simulink model "sgMdl_IO424_LVDTMeasurementTest"  (R2024b)
settings: Solver=FixedStepAuto  StartTime=0.0  StopTime=inf  RelTol=1e-3
model workspace (MAT data in the model file):
  La_ratio = 0.5
libraries: dspsrcs4 x3, speedgoatlib_IO424 x2, speedgoatlib_IO107 x1
Description:
  | IO424 - LVDT Measurement
settings Model: ModifiedByFormat=Speedgoat  SimulationMode=external  ExtModeEnableFloating=off  Creator=Speedgoat  LastModifiedBy=Speedgoat
settings SolverCC: ConcurrentTasks=on  PositivePriorityOrder=on
settings OptimizationCC: BlockReduction=off  OptimizeBlockIOStorage=off
settings DebuggingCC: TasksWithSamePriorityMsg=none
settings HardwareCC: ProdBitPerLong=64  ProdLongLongMode=on  ProdHWDeviceType=Intel->x86-64 (Linux 64)
settings RTWCC: Description=Speedgoat Real-Time Target Machine  SystemTargetFile=speedgoat.tlc  TemplateMakefile=slrealtime_default_tmf  Toolchain=Simulink Real-Time Toolchain  BuildConfiguration=Faster Runs  TargetLang=C++
settings SimulinkRealTimeTargetCC: SubcomponentCodeInterfacePackaging=Reusable function  InstructionSetFMA=off  LogToMDFFile=off  SLRTLogLevel=debug  SLRTFileLogMaxRuns=10
settings ConfigComp: CovBoundaryAbsTol=1.0e-5

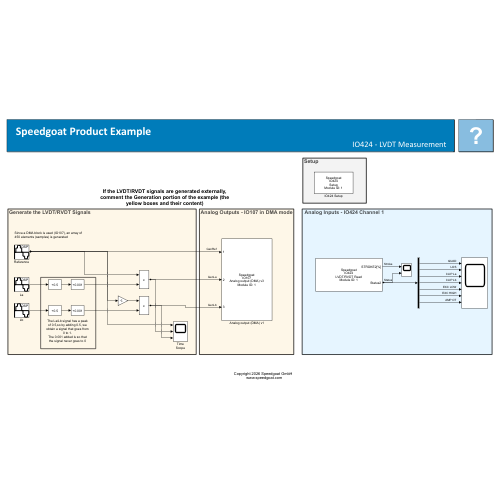
[thumbnail: Simulink's stored preview of the top-level diagram]
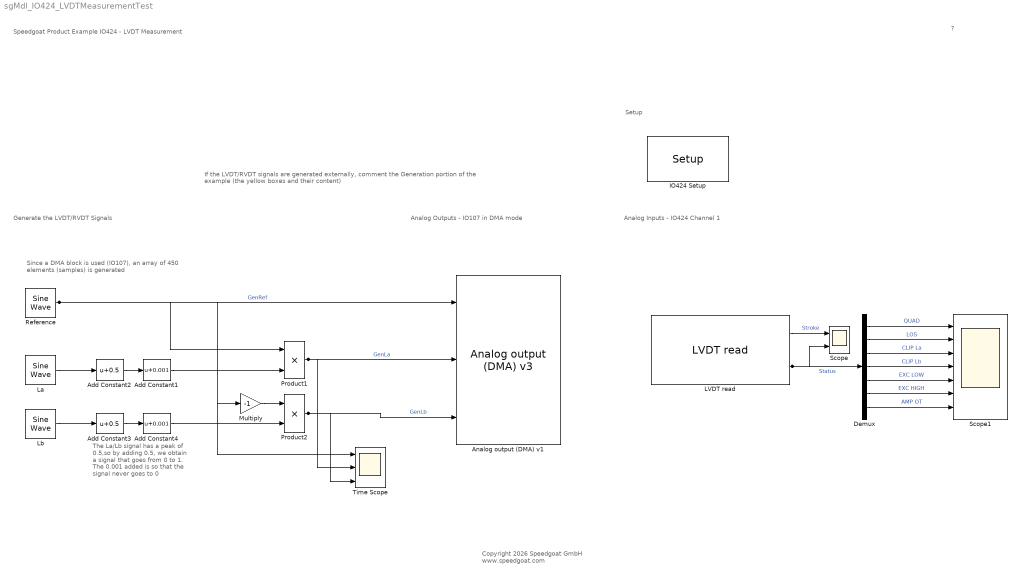
== system sgMdl_IO424_LVDTMeasurementTest ==
  note: The La/Lb signal has a peak
      | of 0.5,so by adding 0.5, we
      | obtain a signal that goes from
      | 0 to 1.
      | The 0.001 added is so that
      | the signal never goes to 0
  note: If the LVDT/RVDT signals are generated externally, comment the Generation portion of the example (the yellow boxes and their content)
  note: Analog Outputs - IO107 in DMA mode
  note: Analog Inputs - IO424 Channel 1
  note: Generate the LVDT/RVDT Signals
  note: Setup
  note: Since a DMA block is used (IO107), an array of
      | 450 elements (samples) is generated
  note: Speedgoat Product Example
      | IO424 - LVDT Measurement
  note: ?
  note: Copyright 2026 Speedgoat GmbH
      |  www.speedgoat.com
  Add Constant1 : Bias  Bias=0.001  SaturateOnIntegerOverflow=off
  Add Constant2 : Bias  Bias=0.5  SaturateOnIntegerOverflow=off
  Add Constant3 : Bias  Bias=0.5  SaturateOnIntegerOverflow=off
  Add Constant4 : Bias  Bias=0.001  SaturateOnIntegerOverflow=off
  Analog output (DMA) v1 : speedgoatlib_IO107/Analog output (DMA) v3  id=1  slot=-1  channel_str=[11 1 10]  range=+-10.0  parInit_str=[0]  parReset_str=[1]  autocal=on  gsense=off  clksrc=Internal  syncmode=Async (replay function)  extsync=LVDS  framesize_str=450  samplerate_str=450e3  sampletime_str=-1
      settings: SourceProductName=IO107
  Demux : Demux  Outputs=7
  IO424 Setup : speedgoatlib_IO424/Setup  parId=1  parModType=IO424-R (no Synchro)  parPciSlot=-1  parChConf1=LVDT/RVDT Ratiometric (6-wires)  parChConf2=Disabled  parChConf3=Disabled  parChConf4=Disabled  parPosRdcUnit=Radiants  parCombRdcCh12=on  parCombRdcCh34=on  parChRdcRange1=7.07 Vrms  parChRdcRange2=14.14 Vrms  parChRdcRange3=14.14 Vrms  parChRdcRange4=14.14 Vrms  parPosSynchroUnit=Radiants  parCombSynchroCh34=on  parChSynchroRange3=28 Vrms  parChSynchroRange4=28 Vrms  parCombLvdtCh12=on  parCombLvdtCh34=on  parLvdtRange1A=7.07 Vrms  parLvdtRange1B=7.07 Vrms  parLvdtRange2A=7.07 Vrms  parLvdtRange2B=14.14 Vrms  parLvdtRange3A=7.07 Vrms  parLvdtRange3B=7.07 Vrms  parLvdtRange4A=7.07 Vrms  parLvdtRange4B=14.14 Vrms  parExcEna1=off  parExcVolt1=2  parExcFreq1=1000  parExcEna2=off  parExcVolt2=2  parExcFreq2=1000  parExcEna3=off  parExcVolt3=2  parExcFreq3=1000  parExcEna4=off  parExcVolt4=2  parExcFreq4=1000
      settings: SourceProductName=IO424
  LVDT read : speedgoatlib_IO424/LVDT read  parId=1  parShowStatus=on  parSampleTime=-1  parChannels=1  parCombCh12=0  parCombCh34=0  parNCh=1
      settings: SourceProductName=IO424
  La : dspsrcs4/Sine Wave  Amplitude=0.5  Frequency=10  Phase=0  SampleMode=Discrete  OutComplex=Real  CompMethod=Trigonometric fcn  TableSize=Speed  SampleTime=1/450e3  SamplesPerFrame=450  ResetState=Restart at time zero  OutputFrames=off  dataType=double  wordLen=16  udDataType=sfix(16)  fracBitsMode=Best precision  numFracBits=15  OutDataTypeStr=double  LastOutDataTypeStr=double
  Lb : dspsrcs4/Sine Wave  Amplitude=0.5  Frequency=10  Phase=pi  SampleMode=Discrete  OutComplex=Real  CompMethod=Trigonometric fcn  TableSize=Speed  SampleTime=1/450e3  SamplesPerFrame=450  ResetState=Restart at time zero  OutputFrames=off  dataType=double  wordLen=16  udDataType=sfix(16)  fracBitsMode=Best precision  numFracBits=15  OutDataTypeStr=double  LastOutDataTypeStr=double
  Multiply : Gain  Gain=-1
  Product1 : Product
  Product2 : Product
  Reference : dspsrcs4/Sine Wave  Amplitude=4*sqrt(2)  Frequency=1e3  Phase=0  SampleMode=Discrete  OutComplex=Real  CompMethod=Trigonometric fcn  TableSize=Speed  SampleTime=1/450e3  SamplesPerFrame=450  ResetState=Restart at time zero  OutputFrames=off  dataType=double  wordLen=16  udDataType=sfix(16)  fracBitsMode=Best precision  numFracBits=15  OutDataTypeStr=double  LastOutDataTypeStr=double
  Scope : Scope  NumInputPorts=2
  Scope1 : Scope  NumInputPorts=7
  Time Scope : Scope  NumInputPorts=3
  wires:
  Add Constant3/1 -> Add Constant4/1
  Multiply/1 -> Product2/1
  LVDT read/1 -> Scope/1  "Stroke"
  La/1 -> Add Constant2/1
  Lb/1 -> Add Constant3/1
  Add Constant4/1 -> Product2/2
  Product1/1 -> Time Scope/2, Analog output (DMA) v1/2  "GenLa"
  Product2/1 -> Time Scope/3, Analog output (DMA) v1/3  "GenLb"
  Reference/1 -> Time Scope/1, Analog output (DMA) v1/1, Multiply/1, Product1/1  "GenRef"
  Add Constant2/1 -> Add Constant1/1
  Add Constant1/1 -> Product1/2
  LVDT read/2 -> Scope/2, Demux/1  "Status"
  Demux/1 -> Scope1/1  "QUAD"
  Demux/2 -> Scope1/2  "LOS"
  Demux/3 -> Scope1/3  "CLIP La"
  Demux/4 -> Scope1/4  "CLIP Lb"
  Demux/5 -> Scope1/5  "EXC LOW"
  Demux/6 -> Scope1/6  "EXC HIGH"
  Demux/7 -> Scope1/7  "AMP OT"
